simulink model "verify_HeatPumpStat_mdl"  (R2018b)
settings: Solver=ode45  StartTime=0  StopTime=1800  MaxStep=120  RelTol=1e-3  EnableMultiTasking=on
InitFcn:
  | load('DE_TRY2010_13_averageYear')
undefined symbols (not defined in the file or in its folder): path_carnot
libraries: carnot x3
settings Model: Creator=drhf  LastModifiedBy=drhf
settings DataIOCC: SaveFormat=Array  SignalLoggingSaveFormat=ModelDataLogs
settings OptimizationCC: ExpressionDepthLimit=2147483647  LifeSpan=inf
settings DebuggingCC: UnderspecifiedInitializationDetection=Classic  MergeDetectMultiDrivingBlocksExec=none  SolverPrmCheckMsg=warning  FcnCallInpInsideContextMsg=warning  StateNameClashWarn=warning  SFUnexpectedBacktrackingDiag=warning  SFNoUnconditionalDefaultTransitionDiag=warning  SFExecutionAtInitializationDiag=none
settings HardwareCC: ProdBitPerPointer=32  ProdBitPerSizeT=32  ProdBitPerPtrDiffT=32  ProdLargestAtomicFloat=None  ProdIntDivRoundTo=Undefined  ProdEndianess=Unspecified  ProdWordSize=32  ProdHWDeviceType=32-bit Generic
settings ModelReferenceCC: PropagateSignalLabelsOutOfModel=off
settings SFSimCC: SimUseLocalCustomCode=off
settings RTWCC: RTWUseLocalCustomCode=off
settings CodeAppCC: StateflowObjectComments=on
settings GRTTargetCC: TargetLangStandard=C89/C90 (ANSI)  GeneratePreprocessorConditionals=Disable all  CombineOutputUpdateFcns=off  GRTInterface=on
settings ConfigComp: CovMetricSettings=dw  CovHtmlReporting=on  CovSaveCumulativeToWorkspaceVar=on  CovSaveSingleToWorkspaceVar=on  CovExternalEMLEnable=off

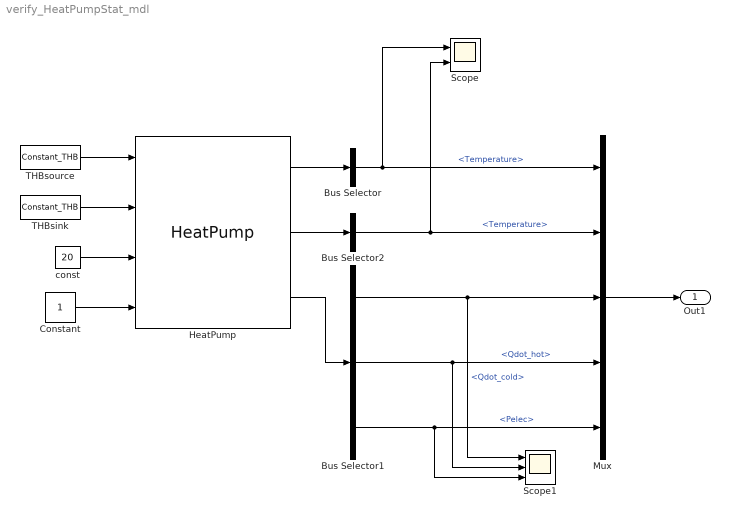
== system verify_HeatPumpStat_mdl ==
  Bus Selector : BusSelector  OutputSignals=Temperature
  Bus Selector1 : BusSelector  OutputSignals=Qdot_cold,Qdot_hot,Pelec
  Bus Selector2 : BusSelector  OutputSignals=Temperature
  Constant : Constant
  HeatPump : carnot/Source/Heat_Pump/HeatPump  PathName=fullfile(path_carnot('libsl'), 'Source', 'Heat_Pump', 'HeatPump', 'parameter_set')  FileName='Vitocal300G_BW106.mat'  userPath=off  userParam=off  K=[172.666667120004 -31.000000610212 7095.00002905086 -6.33333383294697 42.2499995181333 -136.249984347629 178.999999113974 -70.2500000918737 7221.25000248006]  caph=25000  capc=16000  UA=5  relQdotMin=1  linc=10  quac=100  linh=10  quah=100
      settings: SourceProductName=Carnot
  Mux : Mux  Inputs=5
  Scope : Scope  NumInputPorts=2
  Scope1 : Scope  NumInputPorts=3
  THBsink : carnot/Source/Simple/Constant_THB  t=55  mdot=2000/3600  p=1e5  mID=No Pressure Drop  fluid=Water  mix=0  mix2=0  mix3=0  dia=0.02  hgt=0
      settings: SourceProductName=Carnot
  THBsource : carnot/Source/Simple/Constant_THB  t=15  mdot=2000/3600  p=1e5  mID=No Pressure Drop  fluid=Water-Glycol Mix  mix=0.3  mix2=0  mix3=0  dia=0.02  hgt=0
      settings: SourceProductName=Carnot
  const : Constant  Value=20
  Out1 : Outport
  wires:
  HeatPump/1 -> Bus Selector/1
  THBsink/1 -> HeatPump/2
  Bus Selector/1 -> Mux/1, Scope/1  "<Temperature>"
  HeatPump/2 -> Bus Selector2/1
  const/1 -> HeatPump/3
  Constant/1 -> HeatPump/4
  THBsource/1 -> HeatPump/1
  HeatPump/3 -> Bus Selector1/1
  Bus Selector2/1 -> Mux/2, Scope/2  "<Temperature>"
  Bus Selector1/3 -> Mux/5, Scope1/3  "<Pelec>"
  Bus Selector1/2 -> Mux/4, Scope1/2  "<Qdot_hot>"
  Bus Selector1/1 -> Mux/3, Scope1/1  "<Qdot_cold>"
  Mux/1 -> Out1/1
